simulink model "PositionCtrl_nc"  (R2022b)
settings: Solver=VariableStepAuto  StartTime=0.0  StopTime=10.0  RelTol=1e-3
PostLoadFcn:
  | load("lbr14.mat");
libraries: robotmaniplib x1
settings Model: Creator=estek  LastModifiedBy=estek
settings DebuggingCC: UnderSpecifiedDimensionMsg=warning

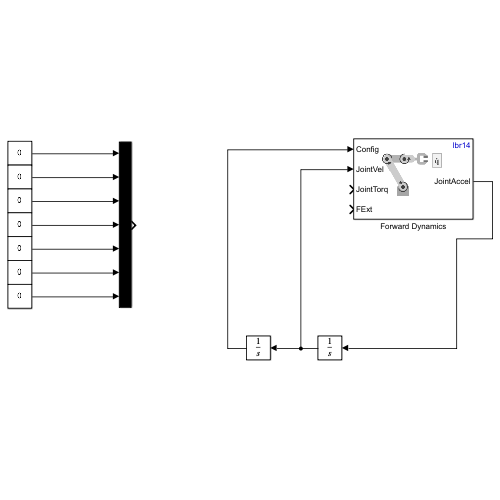
[thumbnail: Simulink's stored preview of the top-level diagram]
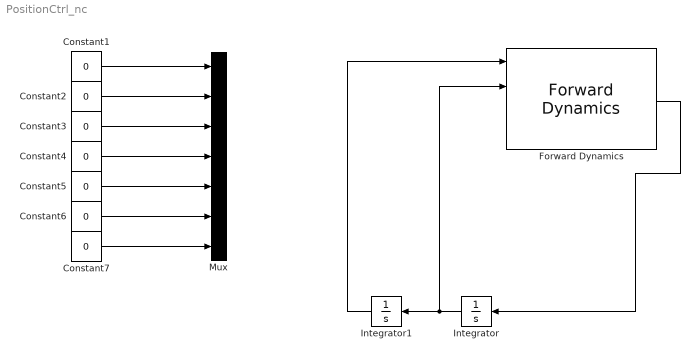
== system PositionCtrl_nc ==
  Constant{1..7} (7 alike) : Constant  Value=0
  Forward Dynamics : robotmaniplib/Forward Dynamics  RigidBodyTree=lbr14  SimulateUsing=Interpreted execution
  Integrator : Integrator
  Integrator1 : Integrator
  Mux : Mux  Inputs=7
  wires:
  Forward Dynamics/1 -> Integrator/1
  Integrator/1 -> Forward Dynamics/2, Integrator1/1
  Integrator1/1 -> Forward Dynamics/1
  Constant1/1 -> Mux/1
  Constant2/1 -> Mux/2
  Constant3/1 -> Mux/3
  Constant4/1 -> Mux/4
  Constant5/1 -> Mux/5
  Constant6/1 -> Mux/6
  Constant7/1 -> Mux/7
